simulink model "problem3"  (R2020b)
settings: Solver=VariableStepAuto  StartTime=0.0  StopTime=10.0  RelTol=1e-3
settings Model: Creator=admin  LastModifiedBy=admin

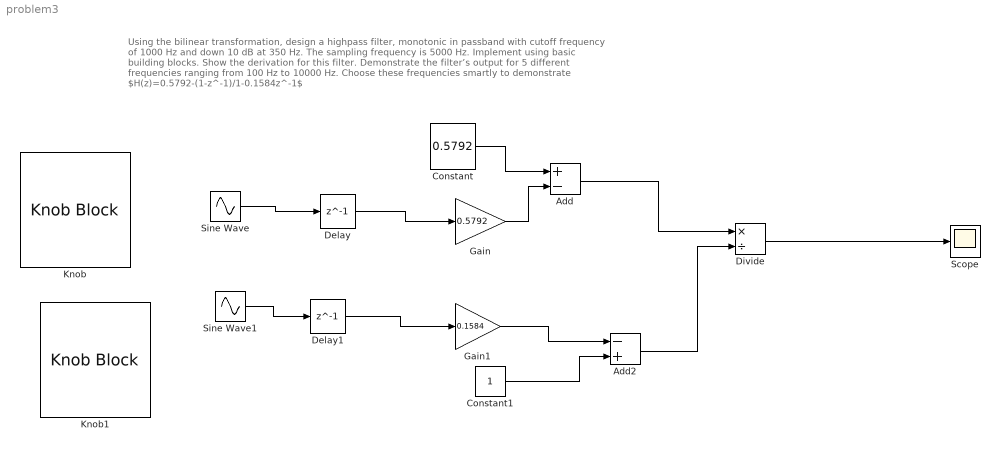
== system problem3 ==
  note: Using the bilinear transformation, design a highpass filter, monotonic in passband with cutoff frequency of 1000 Hz and down 10 dB at 350 Hz. The sampling frequency is 5000 Hz. Implement using basic building blocks. Show the derivation for this filter. Demonstrate the filter’s output for 5 different frequencies ranging from 100 Hz to 10000 Hz. Choose these frequencies smartly to demonstrate $H(z)=0.5792-(1-z^-1)/1-0.1584z^-1$
  Add : Sum  Inputs=+-
  Add2 : Sum  Inputs=-+
  Constant : Constant  Value=0.5792  OutMin=0.5792
  Constant1 : Constant
  Delay : Delay  DelayLength=1
  Delay1 : Delay  DelayLength=1
  Divide : Product  Inputs=*/
  Gain : Gain  Gain=0.5792
  Gain1 : Gain  Gain=0.1584
  Knob : KnobBlock  ScaleMin=100  ScaleMax=1000
  Knob1 : KnobBlock
  Scope : Scope
  Sine Wave : Sin  Frequency=100  SampleTime=0
  Sine Wave1 : Sin  Frequency=100  SampleTime=0
  wires:
  Sine Wave/1 -> Delay/1
  Sine Wave1/1 -> Delay1/1
  Constant/1 -> Add/1
  Delay/1 -> Gain/1
  Gain/1 -> Add/2
  Gain1/1 -> Add2/1
  Delay1/1 -> Gain1/1
  Constant1/1 -> Add2/2
  Add/1 -> Divide/1
  Add2/1 -> Divide/2
  Divide/1 -> Scope/1
